simulink model "Dual_Axis_Solar_Tracker"  (R2022a)
settings: Solver=ode1be  StartTime=0.0  StopTime=121  FixedStep=0.1  MaxStep=1.206E-17  MinStep=1.206E-17  RelTol=1e-5
InitFcn:
  | clear all
  | clc
  | %% PARAMETERS OF DC MOTOR
  | R=18.2214;
  | L=0.000866;
  | Kb=0.030941093;
  | Km=0.030941093;
  | J=0.00009;
  | B1=0.000025;
  | 
  | %% LOADING MPC
  | load mpc1.mat
libraries: mpclib x2
settings Model: Creator=faraj  LastModifiedBy=faraj
settings SolverCC: ExtrapolationOrder=1
settings DataIOCC: SaveOutput=off  SignalLogging=off  DSMLogging=off  SaveTime=off  ReturnWorkspaceOutputs=off
settings ModelReferenceCC: PropagateSignalLabelsOutOfModel=off
settings GRTTargetCC: TargetLangStandard=C89/C90 (ANSI)

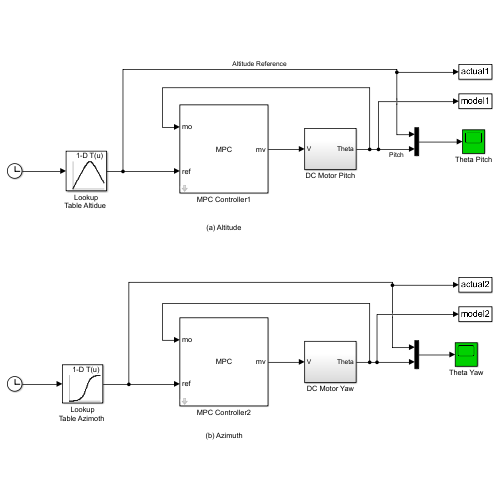
[thumbnail: Simulink's stored preview of the top-level diagram]
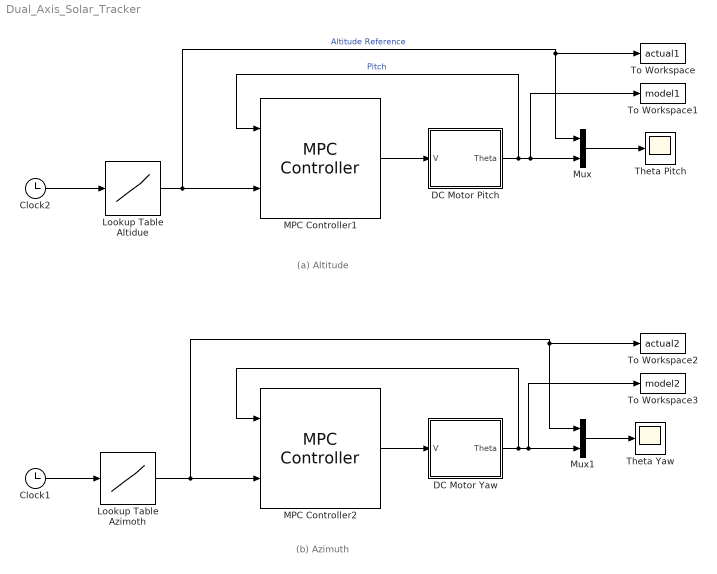
== system Dual_Axis_Solar_Tracker ==
  note: (a) Altitude
  note: (b) Azimuth
  Clock1 : Clock
  Clock2 : Clock
  DC Motor Pitch : Subsystem
  DC Motor Yaw : Subsystem
  "Lookup Table Altidue " : Lookup_n-D  NumberOfTableDimensions=1  BreakpointsForDimension1=[1:121]  BreakpointsForDimension1FirstPoint=0  BreakpointsForDimension1Spacing=0.08264462  Table=|  RndMeth=Simplest
      | [10.21
      | 11.35
      | 12.5
      | 13.64
      | 14.79
      | 15.94
      | 17.08
      | 18.23
      | 19.37
      | 20.52
      | 21.67
      | 22.81
      | 23.96
      | 25.1
      | 26.25
      | 27.39
      | 28.54
      | 29.68
      | 30.82
      | 31.96
      | 33.1
      | 34.24
      | 35.38
      | 36.51
      | 37.64
      | 38.77
      | 39.9
      | 41.03
      | 42.15
      | 43.27
      | 44.39
      | 45.5
      | 46.61
      | 47.72
      | 48.82
      | 49.92
      | 51.01
      | 52.1
      | 53.17
      | 54.25
      | 55.31
      | 56.36
      | 57.41
      | 58.44
      | 59.47
      | 60.48
      | 61.47
      | 62.45
      | 63.42
      | 64.36
      | 65.28
      | 66.18
      | 67.04
      | 67.88
      | 68.69
      | 69.45
      | 70.17
      | 70.85
      | 71.47
      | 72.03
      | 72.53
      | 72.95
      | 73.31
      | 73.58
      | 73.77
      | 73.87
      | 73.88
      | 73.8
      | 73.63
      | 73.38
      | 73.05
      | 72.64
      | 72.16
      | 71.61
      | 71.01
      | 70.35
      | 69.64
      | 68.88
      | 68.09
      | 67.26
      | 66.4
      | 65.51
      | 64.59
      | 63.66
      | 62.7
      | 61.72
      | 60.73
      | 59.72
      | 58.7
      | 57.67
      | 56.63
      | 55.57
      | 54.51
      | 53.44
      | 52.37
      | 51.28
      | 50.19
      | 49.1
      | 48
      | 46.89
      | 45.78
      | 44.67
      | 43.55
      | 42.43
      | 41.31
      | 40.19
      | 39.06
      | 37.93
      | 36.8
      | 35.66
      | 34.52
      | 33.39
      | 32.25
      | 31.11
      | 29.97
      | 28.82
      | 27.68
      | 26.54
      | 25.39
      | 24.25
      | 23.1
      | ]
  "Lookup Table Azimoth " : Lookup_n-D  NumberOfTableDimensions=1  BreakpointsForDimension1=[1:121]  BreakpointsForDimension1FirstPoint=0  BreakpointsForDimension1Spacing=0.08264462  Table=|  RndMeth=Simplest
      | [112.6
      | 112.53
      | 112.47
      | 112.42
      | 112.38
      | 112.35
      | 112.33
      | 112.32
      | 112.32
      | 112.34
      | 112.36
      | 112.39
      | 112.44
      | 112.5
      | 112.56
      | 112.65
      | 112.74
      | 112.85
      | 112.97
      | 113.11
      | 113.26
      | 113.43
      | 113.61
      | 113.82
      | 114.04
      | 114.28
      | 114.54
      | 114.82
      | 115.13
      | 115.45
      | 115.81
      | 116.19
      | 116.61
      | 117.05
      | 117.53
      | 118.04
      | 118.6
      | 119.19
      | 119.83
      | 120.52
      | 121.26
      | 122.06
      | 122.93
      | 123.85
      | 124.86
      | 125.94
      | 127.11
      | 128.38
      | 129.75
      | 131.23
      | 132.83
      | 134.57
      | 136.46
      | 138.5
      | 140.71
      | 143.11
      | 145.69
      | 148.47
      | 151.45
      | 154.65
      | 158.04
      | 161.63
      | 165.39
      | 169.3
      | 173.32
      | 177.42
      | 181.55
      | 185.66
      | 189.7
      | 193.65
      | 197.45
      | 201.08
      | 204.52
      | 207.77
      | 210.8
      | 213.64
      | 216.27
      | 218.7
      | 220.96
      | 223.04
      | 224.97
      | 226.74
      | 228.38
      | 229.9
      | 231.29
      | 232.58
      | 233.78
      | 234.88
      | 235.9
      | 236.85
      | 237.73
      | 238.54
      | 239.3
      | 240
      | 240.66
      | 241.26
      | 241.83
      | 242.35
      | 242.84
      | 243.29
      | 243.71
      | 244.1
      | 244.46
      | 244.8
      | 245.11
      | 245.4
      | 245.66
      | 245.91
      | 246.13
      | 246.34
      | 246.53
      | 246.7
      | 246.86
      | 247
      | 247.13
      | 247.24
      | 247.34
      | 247.42
      | 247.49
      | 247.55
      | 247.6
      | ]
  MPC Controller1 : mpclib/MPC Controller  SCDEnableBlockLinearizationSpecification=on  mpcobj=mpc1  is_multiple=0  enable_value=0  return_u0=off  updateMPCinCallerWorkspace=on  md_inport=off  mv_inport=off  uref_inport=off  return_cost=off  return_mvseq=off  return_qpstatus=off  return_xseq=off  return_state=off  return_ovseq=off  state_inport=off  umin_inport=off  umax_inport=off  ymin_inport=off  ymax_inport=off  cc_inport=off  ywt_inport=off  uwt_inport=off  duwt_inport=off  rhoeps_inport=off  pm_inport=off  MaximumP=10  HorizonChoice=FixedHorizon  n_ts=0.1  n_p=10  n_mv=1  n_md=0  n_ud=0  n_mo=1  n_uo=0  BlockDataType=double  SampleTimeInherited=off  switch_inport=off
  MPC Controller2 : mpclib/MPC Controller  SCDEnableBlockLinearizationSpecification=on  mpcobj=mpc1  is_multiple=0  enable_value=0  return_u0=off  updateMPCinCallerWorkspace=on  md_inport=off  mv_inport=off  uref_inport=off  return_cost=off  return_mvseq=off  return_qpstatus=off  return_xseq=off  return_state=off  return_ovseq=off  state_inport=off  umin_inport=off  umax_inport=off  ymin_inport=off  ymax_inport=off  cc_inport=off  ywt_inport=off  uwt_inport=off  duwt_inport=off  rhoeps_inport=off  pm_inport=off  MaximumP=10  HorizonChoice=FixedHorizon  n_ts=0.1  n_p=10  n_mv=1  n_md=0  n_ud=0  n_mo=1  n_uo=0  BlockDataType=double  SampleTimeInherited=off  switch_inport=off
  Mux : Mux  Inputs=2
  Mux1 : Mux  Inputs=2
  Theta Pitch : Scope
  Theta Yaw : Scope
  To Workspace : ToWorkspace  VariableName=actual1  SampleTime=1
  To Workspace1 : ToWorkspace  VariableName=model1  SampleTime=1
  To Workspace2 : ToWorkspace  VariableName=actual2  SampleTime=1
  To Workspace3 : ToWorkspace  VariableName=model2  SampleTime=1
  wires:
  Clock2/1 -> "Lookup Table Altidue "/1
  "Lookup Table Altidue "/1 -> MPC Controller1/2, Mux/1, To Workspace/1  "Altitude Reference"
  DC Motor Pitch/1(Theta) -> MPC Controller1/1, To Workspace1/1, Mux/2  "Pitch"
  Clock1/1 -> "Lookup Table Azimoth "/1
  MPC Controller2/1 -> DC Motor Yaw/1(V)
  MPC Controller1/1 -> DC Motor Pitch/1(V)
  Mux/1 -> Theta Pitch/1
  Mux1/1 -> Theta Yaw/1
  DC Motor Yaw/1(Theta) -> MPC Controller2/1, To Workspace3/1, Mux1/2
  "Lookup Table Azimoth "/1 -> To Workspace2/1, Mux1/1, MPC Controller2/2

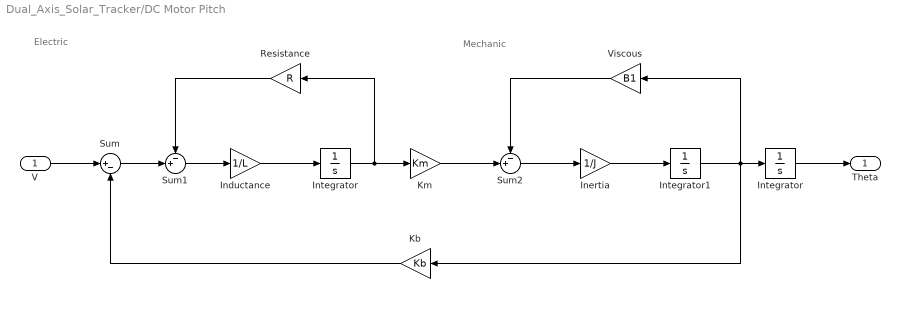
== system Dual_Axis_Solar_Tracker/DC Motor Pitch ==
  note: Mechanic
  note: Electric
  V : Inport
  Inductance : Gain  Gain=1/L
  Inertia : Gain  Gain=1/J
  Integrator : Integrator
  "Integrator " : Integrator
  Integrator1 : Integrator
  Kb : Gain  Gain=Kb
  Km : Gain  Gain=Km
  Resistance : Gain  Gain=R
  Sum : Sum  Inputs=|+-
  Sum1 : Sum  Inputs=-+|
  Sum2 : Sum  Inputs=-+|
  Viscous : Gain  Gain=B1
  Theta : Outport
  wires:
  Km/1 -> Sum2/2
  Kb/1 -> Sum/2
  Inductance/1 -> Integrator/1
  Sum2/1 -> Inertia/1
  Integrator/1 -> Resistance/1, Km/1
  Integrator1/1 -> Kb/1, Viscous/1, "Integrator "/1
  Sum/1 -> Sum1/2
  Sum1/1 -> Inductance/1
  Viscous/1 -> Sum2/1
  Inertia/1 -> Integrator1/1
  Resistance/1 -> Sum1/1
  V/1 -> Sum/1
  "Integrator "/1 -> Theta/1

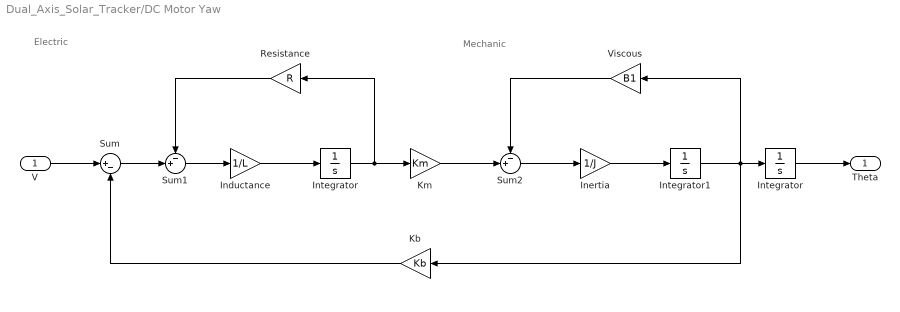
== system Dual_Axis_Solar_Tracker/DC Motor Yaw ==
  note: Mechanic
  note: Electric
  V : Inport
  Inductance : Gain  Gain=1/L
  Inertia : Gain  Gain=1/J
  Integrator : Integrator
  "Integrator " : Integrator
  Integrator1 : Integrator
  Kb : Gain  Gain=Kb
  Km : Gain  Gain=Km
  Resistance : Gain  Gain=R
  Sum : Sum  Inputs=|+-
  Sum1 : Sum  Inputs=-+|
  Sum2 : Sum  Inputs=-+|
  Viscous : Gain  Gain=B1
  Theta : Outport
  wires:
  Km/1 -> Sum2/2
  Kb/1 -> Sum/2
  Inductance/1 -> Integrator/1
  Sum2/1 -> Inertia/1
  Integrator/1 -> Resistance/1, Km/1
  Integrator1/1 -> Kb/1, Viscous/1, "Integrator "/1
  Sum/1 -> Sum1/2
  Sum1/1 -> Inductance/1
  Viscous/1 -> Sum2/1
  Inertia/1 -> Integrator1/1
  Resistance/1 -> Sum1/1
  V/1 -> Sum/1
  "Integrator "/1 -> Theta/1
